simulink model "BANSHEE"  (Simulink 8.1)
settings: Solver=ode1  StartTime=0.0  StopTime=inf  FixedStep=Ts  MaxStep=1e-3  RelTol=1e-3
PostLoadFcn:
  | BANSHEE_init;
InitFcn:
  | BANSHEE_init;
values from neighbouring files (symbols this model uses):
  Ts = 100E-6    (= 0.0001)    [BANSHEE_init.m]
undefined symbols (not defined in the file or in its folder): F1, F2, F3, fdesignblkfcn, Feeder1_lib, Feeder2_lib, Feeder3_lib, gcbh, generic_ethernet_cb, Left, relay_housing_lib, SM_UtilityService, SS_F1_RELAY_HOUSING, SS_F2_RELAY_HOUSING, SS_F3_RELAY_HOUSING, SS_Feeder1, SS_Feeder2, SS_Feeder3, type, utility_service_lib, V
libraries: breaker_lib x47, rtio_generic_modbus x43, relay_modbus_lib x42, cables_lib x41, transformer_lib x22, Load_lib x20, artemis x18, powerlib x18, rtio_opalrt_common x15, ssn_lib x15, rtlab x14, simulink x10
(part 5 of 5)

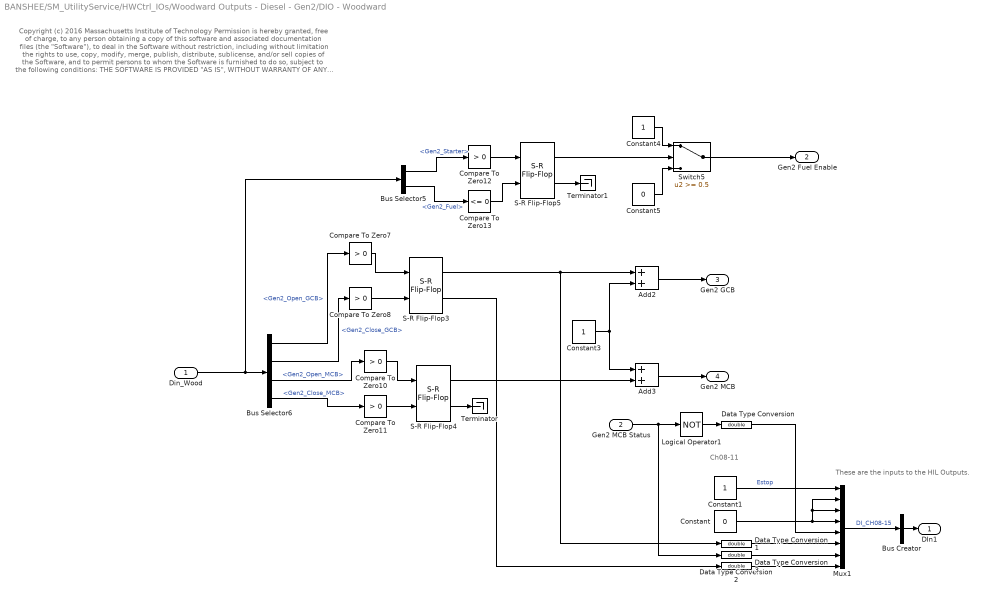
== system BANSHEE/SM_UtilityService/HWCtrl_IOs/Woodward Outputs - Diesel - Gen2/DIO - Woodward ==
  note: Copyright (c) 2016 Massachusetts Institute of Technology
      | Permission is hereby granted, free of charge, to any person obtaining a copy of this software and associated documentation files (the "Software"), to deal
      | in the Software without restriction, including without limitation the rights to use, copy, modify, merge, publish, distribute, sublicense, and/or sell copies of the
      | Software, and to permit persons to whom the Software is furnished to do so, subject to the following conditions:
      |
      | THE SOFTWARE IS PROVIDED "AS IS", WITHOUT WARRANTY OF ANY KIND, EXPRESS OR IMPLIED, INCLUDING BUT NOT LIMITED TO THE
      | WARRANTIES OF MERCHANTABILITY, FITNESS FOR A PARTICULAR PURPOSE AND NONINFRINGEMENT. IN NO EVENT SHALL THE AUTHORS
      | OR COPYRIGHT HOLDERS BE LIABLE FOR ANY CLAIM, DAMAGES OR OTHER LIABILITY, WHETHER IN AN ACTION OF CONTRACT, TORT OR
      | OTHERWISE, ARISING FROM, OUT OF OR IN CONNECTION WITH THE SOFTWARE OR THE USE OR OTHER DEALINGS IN THE SOFTWARE
  note: Ch08-11
  note: These are the inputs to
      | the HIL Outputs.
  Din_Wood : Inport
  Gen2 MCB Status : Inport  Port=2
  Add2 : Sum
  Add3 : Sum
  Bus Creator : BusCreator  Inputs=1
  Bus Selector5 : BusSelector  OutputSignals=DI_CH08-15.Gen2_Starter,DI_CH08-15.Gen2_Fuel
  Bus Selector6 : BusSelector  OutputSignals=DI_CH08-15.Gen2_Open_GCB,DI_CH08-15.Gen2_Close_GCB,DI_CH08-15.Gen2_Open_MCB,DI_CH08-15.Gen2_Close_MCB
  Compare To Zero{7..8,10..12} (5 alike) : simulink/Logic and Bit Operations/Compare To Zero  relop=>  OutDataTypeStr=boolean
  Compare To Zero13 : simulink/Logic and Bit Operations/Compare To Zero  relop=<=  OutDataTypeStr=boolean
  Constant : Constant  Value=0
  Constant1 : Constant
  Constant3 : Constant
  Constant4 : Constant
  Constant5 : Constant  Value=0
  Data Type Conversion{,1..3} (4 alike) : DataTypeConversion  OutDataTypeStr=double
  Logical Operator1 : Logic  Operator=NOT  AllPortsSameDT=off  OutDataTypeStr=boolean
  Mux1 : Mux  Inputs=8
  S-R Flip-Flop3 : simulink_extras/Flip Flops/S-R Flip-Flop  initial_condition=1
  S-R Flip-Flop4 : simulink_extras/Flip Flops/S-R Flip-Flop  initial_condition=1
  S-R Flip-Flop5 : simulink_extras/Flip Flops/S-R Flip-Flop  initial_condition=0
  Switch5 : Switch  Threshold=0.5
  Terminator : Terminator
  Terminator1 : Terminator
  DIn1 : Outport
  Gen2 Fuel Enable : Outport  Port=2
  Gen2 GCB : Outport  Port=3
  Gen2 MCB : Outport  Port=4
  wires:
  Constant1/1 -> Mux1/1  "Estop"
  Data Type Conversion3/1 -> Mux1/8
  Data Type Conversion2/1 -> Mux1/7
  Data Type Conversion1/1 -> Mux1/6
  Constant/1 -> Mux1/4, Mux1/3, Mux1/2
  S-R Flip-Flop5/2 -> Terminator1/1
  S-R Flip-Flop4/2 -> Terminator/1
  Din_Wood/1 -> Bus Selector5/1, Bus Selector6/1
  Bus Creator/1 -> DIn1/1
  Mux1/1 -> Bus Creator/1  "DI_CH08-15"
  S-R Flip-Flop3/1 -> Data Type Conversion1/1, Add2/1
  Bus Selector6/1 -> Compare To Zero7/1  "<Gen2_Open_GCB>"
  Compare To Zero7/1 -> S-R Flip-Flop3/1
  Compare To Zero8/1 -> S-R Flip-Flop3/2
  Bus Selector6/4 -> Compare To Zero11/1  "<Gen2_Close_MCB>"
  Compare To Zero11/1 -> S-R Flip-Flop4/2
  Bus Selector6/3 -> Compare To Zero10/1  "<Gen2_Open_MCB>"
  Compare To Zero10/1 -> S-R Flip-Flop4/1
  Bus Selector6/2 -> Compare To Zero8/1  "<Gen2_Close_GCB>"
  S-R Flip-Flop4/1 -> Add3/2
  Add2/1 -> Gen2 GCB/1
  Add3/1 -> Gen2 MCB/1
  Constant3/1 -> Add2/2, Add3/1
  Bus Selector5/1 -> Compare To Zero12/1  "<Gen2_Starter>"
  Bus Selector5/2 -> Compare To Zero13/1  "<Gen2_Fuel>"
  S-R Flip-Flop5/1 -> Switch5/2
  Compare To Zero12/1 -> S-R Flip-Flop5/1
  Constant5/1 -> Switch5/3
  Constant4/1 -> Switch5/1
  Compare To Zero13/1 -> S-R Flip-Flop5/2
  Switch5/1 -> Gen2 Fuel Enable/1
  Gen2 MCB Status/1 -> Logical Operator1/1, Data Type Conversion2/1
  S-R Flip-Flop3/2 -> Data Type Conversion3/1
  Logical Operator1/1 -> Data Type Conversion/1
  Data Type Conversion/1 -> Mux1/5

== system BANSHEE/SM_UtilityService/HWCtrl_IOs/Woodward Outputs - Diesel - Gen2/DOUT type config ==
  note: The Constants are used to select Digital Output type:
      | - 0: Time-Stamped Digital Output
      | - 1: Pulse-Width Modulated DIgital Output
  DataIn Send : rtio_opalrt_common/DataIn Send  CtrlName='OpCtrl'  FcnNos=11  width=1  portType=double  checkVersion=off  expectedId=0  expectedVersion=0  opComp=>=
      settings: AttributesFormatString=%<CtrlName>
  DataIn Send1 : rtio_opalrt_common/DataIn Send  CtrlName='OpCtrl'  FcnNos=12  width=1  portType=double  checkVersion=off  expectedId=0  expectedVersion=0  opComp=>=
      settings: AttributesFormatString=%<CtrlName>
  Subsection 3 DOUT type : Constant
  Subsection 4 DOUT type : Constant
  Terminator1 : Terminator
  Terminator2 : Terminator
  wires:
  Subsection 3 DOUT type/1 -> DataIn Send/1
  Subsection 4 DOUT type/1 -> DataIn Send1/1
  DataIn Send1/1 -> Terminator1/1
  DataIn Send/1 -> Terminator2/1

== system BANSHEE/SM_UtilityService/HWCtrl_IOs/Woodward Outputs - Diesel - Gen2/Woodward Primary Inputs - Gen2 ==
  note: Copyright (c) 2016 Massachusetts Institute of Technology
      | Permission is hereby granted, free of charge, to any person obtaining a copy of this software and associated documentation files (the "Software"), to deal
      | in the Software without restriction, including without limitation the rights to use, copy, modify, merge, publish, distribute, sublicense, and/or sell copies of the
      | Software, and to permit persons to whom the Software is furnished to do so, subject to the following conditions:
      |
      | THE SOFTWARE IS PROVIDED "AS IS", WITHOUT WARRANTY OF ANY KIND, EXPRESS OR IMPLIED, INCLUDING BUT NOT LIMITED TO THE
      | WARRANTIES OF MERCHANTABILITY, FITNESS FOR A PARTICULAR PURPOSE AND NONINFRINGEMENT. IN NO EVENT SHALL THE AUTHORS
      | OR COPYRIGHT HOLDERS BE LIABLE FOR ANY CLAIM, DAMAGES OR OTHER LIABILITY, WHETHER IN AN ACTION OF CONTRACT, TORT OR
      | OTHERWISE, ARISING FROM, OUT OF OR IN CONNECTION WITH THE SOFTWARE OR THE USE OR OTHER DEALINGS IN THE SOFTWARE
  note: Diesel -> Gen2
  WoodwardBias : Inport
  Bus Creator1 : BusCreator
  Bus Selector5 : BusSelector  OutputSignals=gen2_GOV_bias,gen2_AVR_bias
  Constant8 : Constant  Value=0
  Constant9 : Constant  Value=0
  Divide2 : Product  Inputs=*/
  Divide3 : Product  Inputs=*/
  Gen2 Ref AVR : Constant  Value=1.00
  Gen2 Ref GOV : Constant  Value=1.00
  Lowpass Filter2 : Subsystem  DialogController=fdesignblkfcn  DialogControllerArgs=DataTag2  InitFcn=fdesignblkfcn(gcbh, {'InitFcn'});  mask(Lowpass Filter){}
      mask help: Design a lowpass filter
      settings: CopyFcn=fdesignblkfcn(gcbh, {'CopyFcn'});
      mask Help: helpview(mapfilelocation('dsp'), 'dsplowpassfilter');
      mask Display: disp('Lowpass')
  Lowpass Filter3 : Subsystem  DialogController=fdesignblkfcn  DialogControllerArgs=DataTag4  InitFcn=fdesignblkfcn(gcbh, {'InitFcn'});  mask(Lowpass Filter){}
      mask help: Design a lowpass filter
      settings: CopyFcn=fdesignblkfcn(gcbh, {'CopyFcn'});
      mask Help: helpview(mapfilelocation('dsp'), 'dsplowpassfilter');
      mask Display: disp('Lowpass')
  ScalingBias : Constant  Value=20
  SimulatedBiasValues : Constant  Value=0
  Sum2 : Sum  Inputs=|+-
  Sum3 : Sum  Inputs=|+-
  Switch2 : Switch  Threshold=0.5
  Switch3 : Switch  Threshold=0.5
  bias_enable_for_woodward_ctrl : Constant
  Gen2 Gov and AVR : Outport
  wires:
  bias_enable_for_woodward_ctrl/1 -> Switch2/2, Switch3/2
  ScalingBias/1 -> Divide2/2, Divide3/2
  Divide2/1 -> Sum2/1
  Divide3/1 -> Sum3/1
  Constant8/1 -> Sum2/2
  Constant9/1 -> Sum3/2
  Sum2/1 -> Lowpass Filter2/1(In)
  Switch2/1 -> Bus Creator1/3  "Gen2 GOV"
  Switch3/1 -> Bus Creator1/4  "Gen2 AVR"
  Sum3/1 -> Lowpass Filter3/1(In)
  SimulatedBiasValues/1 -> Switch2/3, Switch3/3
  Lowpass Filter2/1(Out) -> Switch2/1
  Lowpass Filter3/1(Out) -> Switch3/1
  Gen2 Ref AVR/1 -> Bus Creator1/2  "Gen2 Ref AVR"
  Gen2 Ref GOV/1 -> Bus Creator1/1  "Gen2 Ref GOV"
  Bus Creator1/1 -> Gen2 Gov and AVR/1
  WoodwardBias/1 -> Bus Selector5/1
  Bus Selector5/1 -> Divide2/1  "<gen2_GOV_bias>"
  Bus Selector5/2 -> Divide3/1  "<gen2_AVR_bias>"

== system BANSHEE/SM_UtilityService/HWCtrl_IOs/Woodward Outputs - NGCHP - Gen1/DIO - Gr3 ==
  Dout : Inport
  Bus Creator : BusCreator  Inputs=1
  Bus Selector : BusSelector  OutputSignals=DI_CH00-07  OutputAsBus=on
  Conditioning : Subsystem
  DigitalIn : rtio_opalrt_common/DigitalIn  CtrlName='OpCtrl'  portNb=5  FcnNos=Slot 3 Module A Subsection 1  size=1  maxcount=8  count=8  sampleTime=0  numchan=8
      settings: AttributesFormatString=%<CtrlName>
  DigitalOut : rtio_opalrt_common/DigitalOut  CtrlName='OpCtrl'  portNb=5  FcnNos=Slot 3 Module B Subsection 1  size=1  maxcount=8  count=8  numchan=8
      settings: AttributesFormatString=%<CtrlName>
  Terminator3 : Terminator
  Terminator5 : Terminator
  DIn : Outport
  wires:
  DigitalOut/1 -> Terminator3/1
  Dout/1 -> Bus Selector/1
  Bus Selector/1 -> DigitalOut/1
  DigitalIn/2 -> Terminator5/1
  DigitalIn/1 -> Conditioning/1(In1)  "DI_CH00-07"
  Bus Creator/1 -> DIn/1
  Conditioning/1(Out1) -> Bus Creator/1

== system BANSHEE/SM_UtilityService/HWCtrl_IOs/Woodward Outputs - NGCHP - Gen1/DIO - Woodward ==
  note: These are the inputs to
      | the HIL Outputs.
  note: Ch00-03
  note: Copyright (c) 2016 Massachusetts Institute of Technology
      | Permission is hereby granted, free of charge, to any person obtaining a copy of this software and associated documentation files (the "Software"), to deal
      | in the Software without restriction, including without limitation the rights to use, copy, modify, merge, publish, distribute, sublicense, and/or sell copies of the
      | Software, and to permit persons to whom the Software is furnished to do so, subject to the following conditions:
      |
      | THE SOFTWARE IS PROVIDED "AS IS", WITHOUT WARRANTY OF ANY KIND, EXPRESS OR IMPLIED, INCLUDING BUT NOT LIMITED TO THE
      | WARRANTIES OF MERCHANTABILITY, FITNESS FOR A PARTICULAR PURPOSE AND NONINFRINGEMENT. IN NO EVENT SHALL THE AUTHORS
      | OR COPYRIGHT HOLDERS BE LIABLE FOR ANY CLAIM, DAMAGES OR OTHER LIABILITY, WHETHER IN AN ACTION OF CONTRACT, TORT OR
      | OTHERWISE, ARISING FROM, OUT OF OR IN CONNECTION WITH THE SOFTWARE OR THE USE OR OTHER DEALINGS IN THE SOFTWARE
  Din_Wood : Inport
  Gen1 MCB Status : Inport  Port=2
  Add : Sum
  Add1 : Sum
  Bus Creator : BusCreator  Inputs=1
  Bus Selector : BusSelector  OutputSignals=DI_CH00-07.Gen1_Starter,DI_CH00-07.Gen1_Fuel
  Bus Selector3 : BusSelector  OutputSignals=DI_CH00-07.Gen1_Open_GCB,DI_CH00-07.Gen1_Close_GCB,DI_CH00-07.Gen1_Open_MCB,DI_CH00-07.Gen1_Close_MCB
  Compare To Zero{,1,3..4} (4 alike) : simulink/Logic and Bit Operations/Compare To Zero  relop=>  OutDataTypeStr=boolean
  Constant : Constant
  Constant1 : Constant
  Constant3 : Constant  Value=0
  Data Type Conversion{,1..3} (4 alike) : DataTypeConversion  OutDataTypeStr=double
  Data Type Conversion4 : DataTypeConversion
  Logical Operator : Logic  Operator=NOT  AllPortsSameDT=off  OutDataTypeStr=boolean
  Logical Operator2 : Logic  Operator=NOR  AllPortsSameDT=off  OutDataTypeStr=boolean
  Mux2 : Mux  Inputs=8
  S-R Flip-Flop : simulink_extras/Flip Flops/S-R Flip-Flop  initial_condition=1
  S-R Flip-Flop1 : simulink_extras/Flip Flops/S-R Flip-Flop  initial_condition=1
  Terminator : Terminator
  Gen1 Fuel Enable : Outport
  Gen1 GCB : Outport  Port=2
  Gen1 MCB : Outport  Port=3
  DIn1 : Outport  Port=4
  wires:
  Constant1/1 -> Mux2/1  "Estop"
  Data Type Conversion4/1 -> Gen1 Fuel Enable/1
  Bus Selector3/2 -> Compare To Zero1/1  "<Gen1_Close_GCB>"
  Bus Selector3/1 -> Compare To Zero/1  "<Gen1_Open_GCB>"
  Din_Wood/1 -> Bus Selector3/1, Bus Selector/1
  Bus Creator/1 -> DIn1/1
  S-R Flip-Flop/1 -> Add/1, Data Type Conversion2/1
  Compare To Zero/1 -> S-R Flip-Flop/1
  Compare To Zero1/1 -> S-R Flip-Flop/2
  Bus Selector3/4 -> Compare To Zero4/1  "<Gen1_Close_MCB>"
  Compare To Zero4/1 -> S-R Flip-Flop1/2
  Compare To Zero3/1 -> S-R Flip-Flop1/1
  S-R Flip-Flop1/1 -> Add1/2
  Add/1 -> Gen1 GCB/1
  Add1/1 -> Gen1 MCB/1
  Constant/1 -> Add/2, Add1/1
  Bus Selector/1 -> Logical Operator2/1  "<Gen1_Starter>"
  Bus Selector/2 -> Logical Operator2/2  "<Gen1_Fuel>"
  Bus Selector3/3 -> Compare To Zero3/1  "<Gen1_Open_MCB>"
  Gen1 MCB Status/1 -> Data Type Conversion1/1, Logical Operator/1
  S-R Flip-Flop/2 -> Data Type Conversion3/1
  Data Type Conversion/1 -> Mux2/5
  Logical Operator/1 -> Data Type Conversion/1
  Logical Operator2/1 -> Data Type Conversion4/1
  Constant3/1 -> Mux2/4, Mux2/3, Mux2/2
  Mux2/1 -> Bus Creator/1  "DI_CH00-07"
  Data Type Conversion3/1 -> Mux2/8
  Data Type Conversion1/1 -> Mux2/7
  Data Type Conversion2/1 -> Mux2/6
  S-R Flip-Flop1/2 -> Terminator/1

== system BANSHEE/SM_UtilityService/HWCtrl_IOs/Woodward Outputs - NGCHP - Gen1/DOUT type config ==
  note: The Constants are used to select Digital Output type:
      | - 0: Time-Stamped Digital Output
      | - 1: Pulse-Width Modulated DIgital Output
  DataIn Send : rtio_opalrt_common/DataIn Send  CtrlName='OpCtrl'  FcnNos=11  width=1  portType=double  checkVersion=off  expectedId=0  expectedVersion=0  opComp=>=
      settings: AttributesFormatString=%<CtrlName>
  DataIn Send1 : rtio_opalrt_common/DataIn Send  CtrlName='OpCtrl'  FcnNos=12  width=1  portType=double  checkVersion=off  expectedId=0  expectedVersion=0  opComp=>=
      settings: AttributesFormatString=%<CtrlName>
  Subsection 3 DOUT type : Constant
  Subsection 4 DOUT type : Constant
  Terminator1 : Terminator
  Terminator2 : Terminator
  wires:
  Subsection 3 DOUT type/1 -> DataIn Send/1
  Subsection 4 DOUT type/1 -> DataIn Send1/1
  DataIn Send1/1 -> Terminator1/1
  DataIn Send/1 -> Terminator2/1

== system BANSHEE/SM_UtilityService/HWCtrl_IOs/Woodward Outputs - NGCHP - Gen1/Woodward Primary Inputs - Gen1 ==
  note: NG-CHP -> Gen1
  note: Copyright (c) 2016 Massachusetts Institute of Technology
      | Permission is hereby granted, free of charge, to any person obtaining a copy of this software and associated documentation files (the "Software"), to deal
      | in the Software without restriction, including without limitation the rights to use, copy, modify, merge, publish, distribute, sublicense, and/or sell copies of the
      | Software, and to permit persons to whom the Software is furnished to do so, subject to the following conditions:
      |
      | THE SOFTWARE IS PROVIDED "AS IS", WITHOUT WARRANTY OF ANY KIND, EXPRESS OR IMPLIED, INCLUDING BUT NOT LIMITED TO THE
      | WARRANTIES OF MERCHANTABILITY, FITNESS FOR A PARTICULAR PURPOSE AND NONINFRINGEMENT. IN NO EVENT SHALL THE AUTHORS
      | OR COPYRIGHT HOLDERS BE LIABLE FOR ANY CLAIM, DAMAGES OR OTHER LIABILITY, WHETHER IN AN ACTION OF CONTRACT, TORT OR
      | OTHERWISE, ARISING FROM, OUT OF OR IN CONNECTION WITH THE SOFTWARE OR THE USE OR OTHER DEALINGS IN THE SOFTWARE
  WoodwardBias : Inport
  Bus Creator : BusCreator
  Bus Selector5 : BusSelector  OutputSignals=gen1_GOV_bias,gen1_AVR_bias
  Constant3 : Constant  Value=0
  Constant4 : Constant  Value=0
  Divide : Product  Inputs=*/
  Divide1 : Product  Inputs=*/
  Gen1 Ref AVR : Constant  Value=1.00
  Gen1 Ref GOV : Constant  Value=1.00
  Lowpass Filter : Subsystem  DialogController=fdesignblkfcn  DialogControllerArgs=DataTag6  InitFcn=fdesignblkfcn(gcbh, {'InitFcn'});  mask(Lowpass Filter){}
      mask help: Design a lowpass filter
      settings: CopyFcn=fdesignblkfcn(gcbh, {'CopyFcn'});
      mask Help: helpview(mapfilelocation('dsp'), 'dsplowpassfilter');
      mask Display: disp('Lowpass')
  Lowpass Filter1 : Subsystem  DialogController=fdesignblkfcn  DialogControllerArgs=DataTag8  InitFcn=fdesignblkfcn(gcbh, {'InitFcn'});  mask(Lowpass Filter){}
      mask help: Design a lowpass filter
      settings: CopyFcn=fdesignblkfcn(gcbh, {'CopyFcn'});
      mask Help: helpview(mapfilelocation('dsp'), 'dsplowpassfilter');
      mask Display: disp('Lowpass')
  ScalingBias : Constant  Value=20
  SimulatedBiasValues : Constant  Value=0
  Sum : Sum  Inputs=|+-
  Sum1 : Sum  Inputs=|+-
  Switch : Switch  Threshold=0.5
  Switch1 : Switch  Threshold=0.5
  bias_enable_for_woodward_ctrl : Constant
  Gen1 Gov and AVR : Outport
  wires:
  ScalingBias/1 -> Divide/2, Divide1/2
  Divide/1 -> Sum/1
  Divide1/1 -> Sum1/1
  Constant3/1 -> Sum/2
  Constant4/1 -> Sum1/2
  Sum/1 -> Lowpass Filter/1(In)
  Switch/1 -> Bus Creator/3  "Gen1 Gov"
  Switch1/1 -> Bus Creator/4  "Gen1 AVR"
  Sum1/1 -> Lowpass Filter1/1(In)
  SimulatedBiasValues/1 -> Switch/3, Switch1/3
  bias_enable_for_woodward_ctrl/1 -> Switch1/2, Switch/2
  Lowpass Filter/1(Out) -> Switch/1
  Lowpass Filter1/1(Out) -> Switch1/1
  Gen1 Ref AVR/1 -> Bus Creator/2  "Gen1 Ref AVR"
  Gen1 Ref GOV/1 -> Bus Creator/1  "Gen1 Ref GOV"
  Bus Creator/1 -> Gen1 Gov and AVR/1
  WoodwardBias/1 -> Bus Selector5/1
  Bus Selector5/1 -> Divide/1  "<gen1_GOV_bias>"
  Bus Selector5/2 -> Divide1/1  "<gen1_AVR_bias>"

== system BANSHEE/SM_UtilityService/HWCtrl_IOs/Woodward Outputs - Diesel - Gen2/DIO - Gr3/Conditioning1 ==
  In1 : Inport
  Bus Creator : BusCreator  Inputs=8
  Demux : Demux  Outputs=8
  Out1 : Outport
  wires:
  In1/1 -> Demux/1
  Bus Creator/1 -> Out1/1  "DI_CH08-15"
  Demux/8 -> Bus Creator/8  "Gen2_Alarm_CF"
  Demux/7 -> Bus Creator/7  "Gen2_Alarm_AB"
  Demux/6 -> Bus Creator/6  "Gen2_Open_MCB"
  Demux/5 -> Bus Creator/5  "Gen2_Close_MCB"
  Demux/4 -> Bus Creator/4  "Gen2_Open_GCB"
  Demux/3 -> Bus Creator/3  "Gen2_Close_GCB"
  Demux/2 -> Bus Creator/2  "Gen2_Fuel"
  Demux/1 -> Bus Creator/1  "Gen2_Starter"

== system BANSHEE/SM_UtilityService/HWCtrl_IOs/Woodward Outputs - Diesel - Gen2/Woodward Primary Inputs - Gen2/Lowpass Filter2 ==
  In : Inport
  Generated Filter Block : DiscreteFir  Tag=BlockMethodSubSystem  Coefficients=[0.0069552863617617106 0.014587901014631248 -0.0057896483056441538 -0.056861876528372622 -0.059476680260783142 0.076118200884714562 0.29579154768342669 0.40638624201187618 0.29579154768342669 0.076118200884714562 -0.059476680260783142 -0.056861876528372622 -0.0057896483056441538 0.014587901014631248 0.0069552863617617106]  InputProcessing=Columns as channels (frame based)
  Out : Outport
  wires:
  In/1 -> Generated Filter Block/1
  Generated Filter Block/1 -> Out/1

== system BANSHEE/SM_UtilityService/HWCtrl_IOs/Woodward Outputs - Diesel - Gen2/Woodward Primary Inputs - Gen2/Lowpass Filter3 ==
  In : Inport
  Generated Filter Block : DiscreteFir  Tag=BlockMethodSubSystem  Coefficients=[0.0069552863617617106 0.014587901014631248 -0.0057896483056441538 -0.056861876528372622 -0.059476680260783142 0.076118200884714562 0.29579154768342669 0.40638624201187618 0.29579154768342669 0.076118200884714562 -0.059476680260783142 -0.056861876528372622 -0.0057896483056441538 0.014587901014631248 0.0069552863617617106]  InputProcessing=Columns as channels (frame based)
  Out : Outport
  wires:
  In/1 -> Generated Filter Block/1
  Generated Filter Block/1 -> Out/1

== system BANSHEE/SM_UtilityService/HWCtrl_IOs/Woodward Outputs - NGCHP - Gen1/DIO - Gr3/Conditioning ==
  In1 : Inport
  Bus Creator : BusCreator  Inputs=8
  Demux : Demux  Outputs=8
  Out1 : Outport
  wires:
  Demux/1 -> Bus Creator/1  "Gen1_Starter"
  Demux/2 -> Bus Creator/2  "Gen1_Fuel"
  Demux/3 -> Bus Creator/3  "Gen1_Close_GCB"
  Demux/4 -> Bus Creator/4  "Gen1_Open_GCB"
  Demux/5 -> Bus Creator/5  "Gen1_Close_MCB"
  Demux/6 -> Bus Creator/6  "Gen1_Open_MCB"
  Demux/7 -> Bus Creator/7  "Gen1_Alarm_AB"
  Demux/8 -> Bus Creator/8  "Gen1_Alarm_CF"
  Bus Creator/1 -> Out1/1  "DI_CH00-07"
  In1/1 -> Demux/1

== system BANSHEE/SM_UtilityService/HWCtrl_IOs/Woodward Outputs - NGCHP - Gen1/Woodward Primary Inputs - Gen1/Lowpass Filter ==
  In : Inport
  Generated Filter Block : DiscreteFir  Tag=BlockMethodSubSystem  Coefficients=[0.0069552863617617106 0.014587901014631248 -0.0057896483056441538 -0.056861876528372622 -0.059476680260783142 0.076118200884714562 0.29579154768342669 0.40638624201187618 0.29579154768342669 0.076118200884714562 -0.059476680260783142 -0.056861876528372622 -0.0057896483056441538 0.014587901014631248 0.0069552863617617106]  InputProcessing=Columns as channels (frame based)
  Out : Outport
  wires:
  In/1 -> Generated Filter Block/1
  Generated Filter Block/1 -> Out/1

== system BANSHEE/SM_UtilityService/HWCtrl_IOs/Woodward Outputs - NGCHP - Gen1/Woodward Primary Inputs - Gen1/Lowpass Filter1 ==
  In : Inport
  Generated Filter Block : DiscreteFir  Tag=BlockMethodSubSystem  Coefficients=[0.0069552863617617106 0.014587901014631248 -0.0057896483056441538 -0.056861876528372622 -0.059476680260783142 0.076118200884714562 0.29579154768342669 0.40638624201187618 0.29579154768342669 0.076118200884714562 -0.059476680260783142 -0.056861876528372622 -0.0057896483056441538 0.014587901014631248 0.0069552863617617106]  InputProcessing=Columns as channels (frame based)
  Out : Outport
  wires:
  In/1 -> Generated Filter Block/1
  Generated Filter Block/1 -> Out/1

== matlab function SS_F3_RELAY_HOUSING/Banshee UDP Data - Formatted Packets/Cast uint16 ==
  data: u input double; y output double
function y = fcn(u)
%#codegen

x = double(typecast(uint32(u),'uint16'));
y = x(1); % low bits
